simulink model "quaternionPropagate"  (R2023b)
settings: Solver=VariableStepAuto  StartTime=0.0  StopTime=Tfinal  RelTol=1e-3
model workspace (MAT data in the model file):
  q0 = [-0.0249340053446; 0.0808200282066; -0.258785631278; 0.962224721914]
libraries: vrlib x1
settings Model: Creator=stanforduser  LastModifiedBy=kristopherriordan
settings DataIOCC: ReturnWorkspaceOutputs=off  OutputSaveName=R  OutputOption=SpecifiedOutputTimes  OutputTimes=t

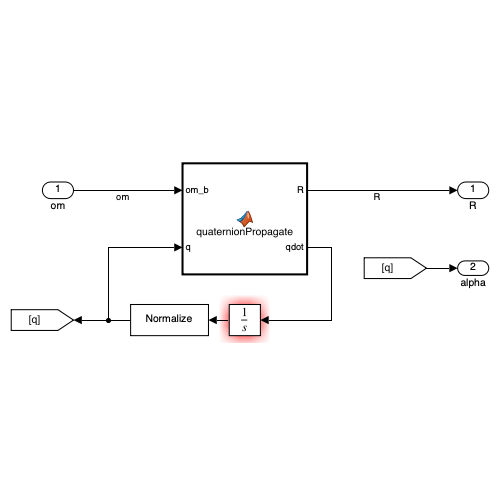
[thumbnail: Simulink's stored preview of the top-level diagram]
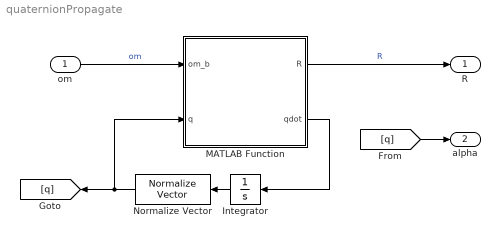
== system quaternionPropagate ==
  om : Inport
  Integrator : Integrator  InitialCondition=q0
  MATLAB Function : MATLAB Function  TreatAsAtomicUnit=on
  Normalize Vector : vrlib/Utilities/Normalize Vector  maxzero=0
  R : Outport
  alpha : Outport  Port=2
  wires:
  om/1 -> MATLAB Function/1(om_b)  "om"
  MATLAB Function/1(R) -> R/1  "R"
  MATLAB Function/2(qdot) -> Integrator/1
  Integrator/1 -> Normalize Vector/1
  Normalize Vector/1 -> MATLAB Function/2(q), [q]
  [q] -> alpha/1

== matlab function quaternionPropagate/MATLAB Function ==
  data: om_b input size=[3 1]; q input; R output; qdot output
function [R, qdot] = quaternionPropagate(om_b, q)

% udot = zeros(size(u));
% q = q./norm(q);
q0 = q(1);
q1 = q(2);
q2 = q(3);
q3 = q(4);
% qvec = q(2:end);

W_prime = [-q1, q0, q3, -q2;
            -q2, -q3, q0, q1;
            -q3, q2, -q1, q0];

qdot = (1/2)*(W_prime.')*om_b;


R = [q0^2 + q1^2 - q2^2 - q3^2, 2*q1*q2 + 2*q0 *q3, 2*(q1*q3 - q0*q2);
    2*(q1*q2 - q0*q3), q0^2 - q1^2 + q2^2 - q3^2, 2*(q2*q3 + q0*q1);
    2*(q1*q3 + q0*q2), 2*(q2*q3 - q0*q1), q0^2 - q1^2 - q2^2 + q3^2];
